simulink model "E33_VCU_simulink"  (R2014a)
settings: Solver=FixedStepDiscrete  StartTime=0.0  StopTime=10.0  FixedStep=0.0005  RelTol=1e-3
values from neighbouring files (symbols this model uses):
  Accu_FAN_Test = ecucoder_cal(Accu_FAN_Test)    [E33_VCU.m]
  Accu_FAN_threshold = ecucoder_cal(Accu_FAN_threshold)    [E33_VCU.m]
  APPS1_Voltage = ecucoder_cal(APPS1_Voltage)    [E33_VCU.m]
  APPS2_Voltage = ecucoder_cal(APPS2_Voltage)    [E33_VCU.m]
  APPS_Map = [0,1000]    [E33_VCU.m]
  APPS_threshold = ecucoder_cal(APPS_threshold)    [E33_VCU.m]
  Beep_Time = ecucoder_cal(Beep_Time)    [E33_VCU.m]
  BeeperTest = ecucoder_cal(BeeperTest)    [E33_VCU.m]
  BMSLedTest = ecucoder_cal(BMSLedTest)    [E33_VCU.m]
  BP_F_threshold = ecucoder_cal(BP_F_threshold)    [E33_VCU.m]
  BP_F_Voltage = ecucoder_cal(BP_F_Voltage)    [E33_VCU.m]
  BP_Map = [0,1000]    [E33_VCU.m]
  BP_R_Voltage = ecucoder_cal(BP_R_Voltage)    [E33_VCU.m]
  Brk_luminance = ecucoder_cal(Brk_luminance)    [E33_VCU.m]
  DCDC_Relay_Test = ecucoder_cal(DCDC_Relay_Test)    [E33_VCU.m]
  FactoryTestEnable = ecucoder_cal(FactoryTestEnable)    [E33_VCU.m]
  HardBrk_luminance = ecucoder_cal(HardBrk_luminance)    [E33_VCU.m]
  IMDLedTest = ecucoder_cal(IMDLedTest)    [E33_VCU.m]
  linear_FL_Map = ecucoder_cal(linear_FL_Map)    [E33_VCU.m]
  linear_FR_Map = ecucoder_cal(linear_FR_Map)    [E33_VCU.m]
  linear_Map = ecucoder_cal(linear_Map)    [E33_VCU.m]
  linear_RL_Map = ecucoder_cal(linear_RL_Map)    [E33_VCU.m]
  linear_RR_Map = ecucoder_cal(linear_RR_Map)    [E33_VCU.m]
  MaxPow = 40    [E33_VCU.m]
  MaxRPM = 5400    [E33_VCU.m]
  MaxRPMchangePerSec = ecucoder_cal(MaxRPMchangePerSec)    [E33_VCU.m]
  MaxTorqChangePerSec = ecucoder_cal(MaxTorqChangePerSec)    [E33_VCU.m]
  Motor_RPM_Map = (0:ceil(MaxRPM/100))*100    [E33_VCU.m]
  Pump_Test = ecucoder_cal(Pump_Test)    [E33_VCU.m]
  Pump_threshold = ecucoder_cal(Pump_threshold)    [E33_VCU.m]
  R2D_Light_Test = ecucoder_cal(R2D_Light_Test)    [E33_VCU.m]
  Radiator_FAN_Test = ecucoder_cal(Radiator_FAN_Test)    [E33_VCU.m]
  SCS_Error_5V = ecucoder_cal(SCS_Error_5V)    [E33_VCU.m]
  SCS_Error_GND = ecucoder_cal(SCS_Error_GND)    [E33_VCU.m]
  SPD_Coef = 1884/40    (= 47.1)    [E33_VCU.m]
  Tail_Light_Test = ecucoder_cal(Tail_Light_Test)    [E33_VCU.m]
  Tmanage_Map = [0,100]    [E33_VCU.m]
  Torq_percentage_Map = Motor_Torq_MAP/MaxTorq*1000    [E33_VCU.m]
libraries: simulink x164, ec55xxlib x44, dspswit3 x6
(part 4 of 5)

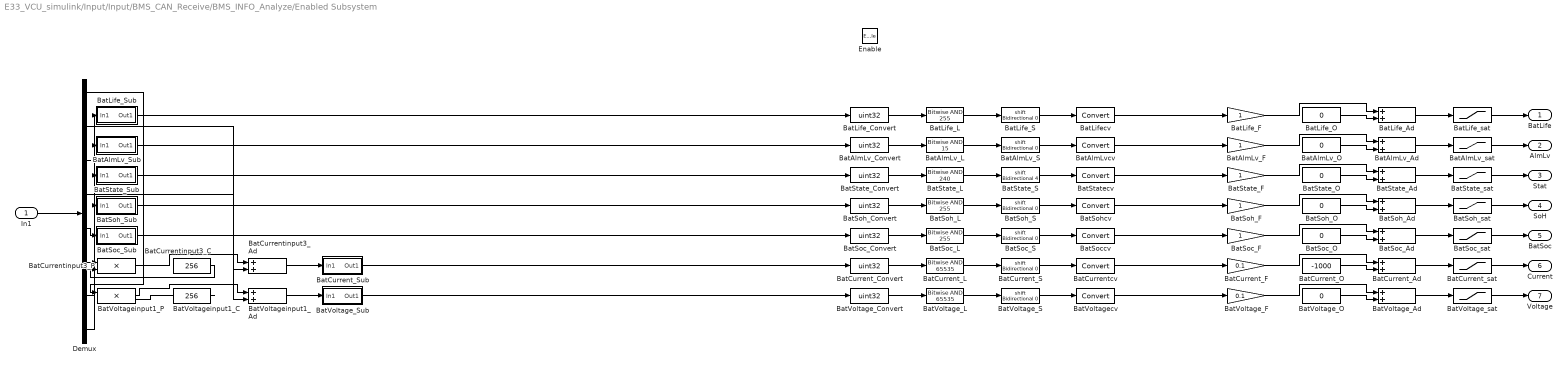
== system E33_VCU_simulink/Input/Input/BMS_CAN_Receive/BMS_INFO_Analyze/Enabled Subsystem ==
  In1 : Inport
  Enable : EnablePort
  BatAlmLv_Ad : Sum
  BatAlmLv_Convert : DataTypeConversion  OutDataTypeStr=uint32
  BatAlmLv_F : Gain
  BatAlmLv_L : simulink/Logic and Bit Operations/Bitwise Operator  logicop=AND  UseBitMask=on  BitMask=15  BitMaskRealWorld=Stored Integer
  BatAlmLv_O : Constant  Value=0  OutDataTypeStr=single
  BatAlmLv_S : ArithShift
  BatAlmLv_Sub : Subsystem
  BatAlmLv_sat : Saturate  UpperLimit=4  LowerLimit=0
  BatAlmLvcv : DataTypeConversion
  BatCurrent_Ad : Sum
  BatCurrent_Convert : DataTypeConversion  OutDataTypeStr=uint32
  BatCurrent_F : Gain  Gain=0.1
  BatCurrent_L : simulink/Logic and Bit Operations/Bitwise Operator  logicop=AND  UseBitMask=on  BitMask=65535  BitMaskRealWorld=Stored Integer
  BatCurrent_O : Constant  Value=-1000  OutDataTypeStr=single
  BatCurrent_S : ArithShift
  BatCurrent_Sub : Subsystem
  BatCurrent_sat : Saturate  UpperLimit=1000  LowerLimit=-1000
  BatCurrentcv : DataTypeConversion
  BatCurrentinput3_Ad : Sum
  BatCurrentinput3_C : Constant  Value=256
  BatCurrentinput3_P : Product
  BatLife_Ad : Sum
  BatLife_Convert : DataTypeConversion  OutDataTypeStr=uint32
  BatLife_F : Gain
  BatLife_L : simulink/Logic and Bit Operations/Bitwise Operator  logicop=AND  UseBitMask=on  BitMask=255  BitMaskRealWorld=Stored Integer
  BatLife_O : Constant  Value=0  OutDataTypeStr=single
  BatLife_S : ArithShift
  BatLife_Sub : Subsystem
  BatLife_sat : Saturate  UpperLimit=255  LowerLimit=0
  BatLifecv : DataTypeConversion
  BatSoc_Ad : Sum
  BatSoc_Convert : DataTypeConversion  OutDataTypeStr=uint32
  BatSoc_F : Gain
  BatSoc_L : simulink/Logic and Bit Operations/Bitwise Operator  logicop=AND  UseBitMask=on  BitMask=255  BitMaskRealWorld=Stored Integer
  BatSoc_O : Constant  Value=0  OutDataTypeStr=single
  BatSoc_S : ArithShift
  BatSoc_Sub : Subsystem
  BatSoc_sat : Saturate  UpperLimit=100  LowerLimit=0
  BatSoccv : DataTypeConversion
  BatSoh_Ad : Sum
  BatSoh_Convert : DataTypeConversion  OutDataTypeStr=uint32
  BatSoh_F : Gain
  BatSoh_L : simulink/Logic and Bit Operations/Bitwise Operator  logicop=AND  UseBitMask=on  BitMask=255  BitMaskRealWorld=Stored Integer
  BatSoh_O : Constant  Value=0  OutDataTypeStr=single
  BatSoh_S : ArithShift
  BatSoh_Sub : Subsystem
  BatSoh_sat : Saturate  UpperLimit=100  LowerLimit=0
  BatSohcv : DataTypeConversion
  BatState_Ad : Sum
  BatState_Convert : DataTypeConversion  OutDataTypeStr=uint32
  BatState_F : Gain
  BatState_L : simulink/Logic and Bit Operations/Bitwise Operator  logicop=AND  UseBitMask=on  BitMask=240  BitMaskRealWorld=Stored Integer
  BatState_O : Constant  Value=0  OutDataTypeStr=single
  BatState_S : ArithShift  BitShiftNumber=4
  BatState_Sub : Subsystem
  BatState_sat : Saturate  UpperLimit=7  LowerLimit=0
  BatStatecv : DataTypeConversion
  BatVoltage_Ad : Sum
  BatVoltage_Convert : DataTypeConversion  OutDataTypeStr=uint32
  BatVoltage_F : Gain  Gain=0.1
  BatVoltage_L : simulink/Logic and Bit Operations/Bitwise Operator  logicop=AND  UseBitMask=on  BitMask=65535  BitMaskRealWorld=Stored Integer
  BatVoltage_O : Constant  Value=0  OutDataTypeStr=single
  BatVoltage_S : ArithShift
  BatVoltage_Sub : Subsystem
  BatVoltage_sat : Saturate  UpperLimit=900  LowerLimit=0
  BatVoltagecv : DataTypeConversion
  BatVoltageinput1_Ad : Sum
  BatVoltageinput1_C : Constant  Value=256
  BatVoltageinput1_P : Product
  Demux : Demux  Outputs=8
  BatLife : Outport
  AlmLv : Outport  Port=2
  Stat : Outport  Port=3
  SoH : Outport  Port=4
  BatSoc : Outport  Port=5
  Current : Outport  Port=6
  Voltage : Outport  Port=7
  wires:
  In1/1 -> Demux/1
  BatVoltagecv/1 -> BatVoltage_F/1
  BatVoltage_S/1 -> BatVoltagecv/1
  BatVoltage_L/1 -> BatVoltage_S/1
  BatVoltage_Convert/1 -> BatVoltage_L/1
  BatVoltage_Sub/1(Out1) -> BatVoltage_Convert/1
  BatVoltageinput1_Ad/1 -> BatVoltage_Sub/1(In1)
  Demux/2 -> BatVoltageinput1_Ad/2
  BatVoltageinput1_P/1 -> BatVoltageinput1_Ad/1
  BatVoltageinput1_C/1 -> BatVoltageinput1_P/2
  Demux/1 -> BatVoltageinput1_P/1
  BatVoltage_sat/1 -> Voltage/1
  BatVoltage_Ad/1 -> BatVoltage_sat/1
  BatVoltage_O/1 -> BatVoltage_Ad/2
  BatVoltage_F/1 -> BatVoltage_Ad/1
  BatCurrentcv/1 -> BatCurrent_F/1
  BatCurrent_S/1 -> BatCurrentcv/1
  BatCurrent_L/1 -> BatCurrent_S/1
  BatCurrent_Convert/1 -> BatCurrent_L/1
  BatCurrent_Sub/1(Out1) -> BatCurrent_Convert/1
  BatCurrentinput3_Ad/1 -> BatCurrent_Sub/1(In1)
  Demux/4 -> BatCurrentinput3_Ad/2
  BatCurrentinput3_P/1 -> BatCurrentinput3_Ad/1
  BatCurrentinput3_C/1 -> BatCurrentinput3_P/2
  Demux/3 -> BatCurrentinput3_P/1
  BatCurrent_sat/1 -> Current/1
  BatCurrent_Ad/1 -> BatCurrent_sat/1
  BatCurrent_O/1 -> BatCurrent_Ad/2
  BatCurrent_F/1 -> BatCurrent_Ad/1
  BatSoccv/1 -> BatSoc_F/1
  BatSoc_S/1 -> BatSoccv/1
  BatSoc_L/1 -> BatSoc_S/1
  BatSoc_Convert/1 -> BatSoc_L/1
  BatSoc_Sub/1(Out1) -> BatSoc_Convert/1
  Demux/5 -> BatSoc_Sub/1(In1)
  BatSoc_sat/1 -> BatSoc/1
  BatSoc_Ad/1 -> BatSoc_sat/1
  BatSoc_O/1 -> BatSoc_Ad/2
  BatSoc_F/1 -> BatSoc_Ad/1
  BatSohcv/1 -> BatSoh_F/1
  BatSoh_S/1 -> BatSohcv/1
  BatSoh_L/1 -> BatSoh_S/1
  BatSoh_Convert/1 -> BatSoh_L/1
  BatSoh_Sub/1(Out1) -> BatSoh_Convert/1
  Demux/6 -> BatSoh_Sub/1(In1)
  BatSoh_sat/1 -> SoH/1
  BatSoh_Ad/1 -> BatSoh_sat/1
  BatSoh_O/1 -> BatSoh_Ad/2
  BatSoh_F/1 -> BatSoh_Ad/1
  BatStatecv/1 -> BatState_F/1
  BatState_S/1 -> BatStatecv/1
  BatState_L/1 -> BatState_S/1
  BatState_Convert/1 -> BatState_L/1
  BatState_Sub/1(Out1) -> BatState_Convert/1
  BatState_sat/1 -> Stat/1
  BatState_Ad/1 -> BatState_sat/1
  BatState_O/1 -> BatState_Ad/2
  BatState_F/1 -> BatState_Ad/1
  BatAlmLvcv/1 -> BatAlmLv_F/1
  BatAlmLv_S/1 -> BatAlmLvcv/1
  BatAlmLv_L/1 -> BatAlmLv_S/1
  BatAlmLv_Convert/1 -> BatAlmLv_L/1
  BatAlmLv_Sub/1(Out1) -> BatAlmLv_Convert/1
  Demux/7 -> BatAlmLv_Sub/1(In1), BatState_Sub/1(In1)
  BatAlmLv_sat/1 -> AlmLv/1
  BatAlmLv_Ad/1 -> BatAlmLv_sat/1
  BatAlmLv_O/1 -> BatAlmLv_Ad/2
  BatAlmLv_F/1 -> BatAlmLv_Ad/1
  BatLifecv/1 -> BatLife_F/1
  BatLife_S/1 -> BatLifecv/1
  BatLife_L/1 -> BatLife_S/1
  BatLife_Convert/1 -> BatLife_L/1
  BatLife_Sub/1(Out1) -> BatLife_Convert/1
  Demux/8 -> BatLife_Sub/1(In1)
  BatLife_sat/1 -> BatLife/1
  BatLife_Ad/1 -> BatLife_sat/1
  BatLife_O/1 -> BatLife_Ad/2
  BatLife_F/1 -> BatLife_Ad/1

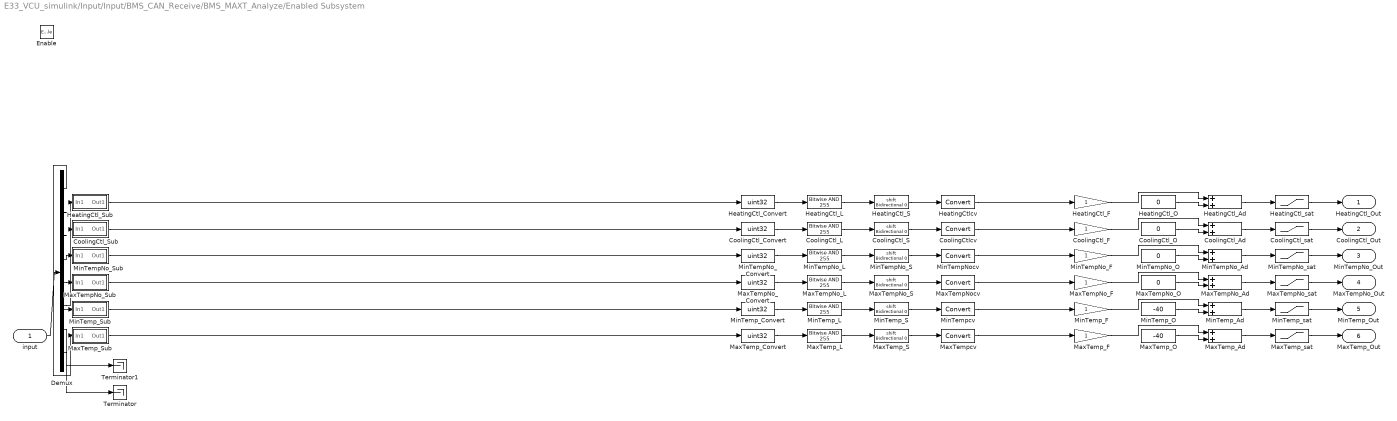
== system E33_VCU_simulink/Input/Input/BMS_CAN_Receive/BMS_MAXT_Analyze/Enabled Subsystem ==
  input : Inport
  Enable : EnablePort
  CoolingCtl_Ad : Sum
  CoolingCtl_Convert : DataTypeConversion  OutDataTypeStr=uint32
  CoolingCtl_F : Gain
  CoolingCtl_L : simulink/Logic and Bit Operations/Bitwise Operator  logicop=AND  UseBitMask=on  BitMask=255  BitMaskRealWorld=Stored Integer
  CoolingCtl_O : Constant  Value=0  OutDataTypeStr=single
  CoolingCtl_S : ArithShift
  CoolingCtl_Sub : Subsystem
  CoolingCtl_sat : Saturate  UpperLimit=1  LowerLimit=0
  CoolingCtlcv : DataTypeConversion
  Demux : Demux  Outputs=8
  HeatingCtl_Ad : Sum
  HeatingCtl_Convert : DataTypeConversion  OutDataTypeStr=uint32
  HeatingCtl_F : Gain
  HeatingCtl_L : simulink/Logic and Bit Operations/Bitwise Operator  logicop=AND  UseBitMask=on  BitMask=255  BitMaskRealWorld=Stored Integer
  HeatingCtl_O : Constant  Value=0  OutDataTypeStr=single
  HeatingCtl_S : ArithShift
  HeatingCtl_Sub : Subsystem
  HeatingCtl_sat : Saturate  UpperLimit=1  LowerLimit=0
  HeatingCtlcv : DataTypeConversion
  MaxTempNo_Ad : Sum
  MaxTempNo_Convert : DataTypeConversion  OutDataTypeStr=uint32
  MaxTempNo_F : Gain
  MaxTempNo_L : simulink/Logic and Bit Operations/Bitwise Operator  logicop=AND  UseBitMask=on  BitMask=255  BitMaskRealWorld=Stored Integer
  MaxTempNo_O : Constant  Value=0  OutDataTypeStr=single
  MaxTempNo_S : ArithShift
  MaxTempNo_Sub : Subsystem
  MaxTempNo_sat : Saturate  UpperLimit=255  LowerLimit=0
  MaxTempNocv : DataTypeConversion
  MaxTemp_Ad : Sum
  MaxTemp_Convert : DataTypeConversion  OutDataTypeStr=uint32
  MaxTemp_F : Gain
  MaxTemp_L : simulink/Logic and Bit Operations/Bitwise Operator  logicop=AND  UseBitMask=on  BitMask=255  BitMaskRealWorld=Stored Integer
  MaxTemp_O : Constant  Value=-40  OutDataTypeStr=single
  MaxTemp_S : ArithShift
  MaxTemp_Sub : Subsystem
  MaxTemp_sat : Saturate  UpperLimit=120  LowerLimit=-40
  MaxTempcv : DataTypeConversion
  MinTempNo_Ad : Sum
  MinTempNo_Convert : DataTypeConversion  OutDataTypeStr=uint32
  MinTempNo_F : Gain
  MinTempNo_L : simulink/Logic and Bit Operations/Bitwise Operator  logicop=AND  UseBitMask=on  BitMask=255  BitMaskRealWorld=Stored Integer
  MinTempNo_O : Constant  Value=0  OutDataTypeStr=single
  MinTempNo_S : ArithShift
  MinTempNo_Sub : Subsystem
  MinTempNo_sat : Saturate  UpperLimit=255  LowerLimit=0
  MinTempNocv : DataTypeConversion
  MinTemp_Ad : Sum
  MinTemp_Convert : DataTypeConversion  OutDataTypeStr=uint32
  MinTemp_F : Gain
  MinTemp_L : simulink/Logic and Bit Operations/Bitwise Operator  logicop=AND  UseBitMask=on  BitMask=255  BitMaskRealWorld=Stored Integer
  MinTemp_O : Constant  Value=-40  OutDataTypeStr=single
  MinTemp_S : ArithShift
  MinTemp_Sub : Subsystem
  MinTemp_sat : Saturate  UpperLimit=120  LowerLimit=-40
  MinTempcv : DataTypeConversion
  Terminator : Terminator
  Terminator1 : Terminator
  HeatingCtl_Out : Outport
  CoolingCtl_Out : Outport  Port=2
  MinTempNo_Out : Outport  Port=3
  MaxTempNo_Out : Outport  Port=4
  MinTemp_Out : Outport  Port=5
  MaxTemp_Out : Outport  Port=6
  wires:
  HeatingCtl_F/1 -> HeatingCtl_Ad/1
  HeatingCtl_O/1 -> HeatingCtl_Ad/2
  HeatingCtl_Ad/1 -> HeatingCtl_sat/1
  HeatingCtl_sat/1 -> HeatingCtl_Out/1
  Demux/6 -> HeatingCtl_Sub/1(In1)
  HeatingCtl_Sub/1(Out1) -> HeatingCtl_Convert/1
  HeatingCtl_Convert/1 -> HeatingCtl_L/1
  HeatingCtl_L/1 -> HeatingCtl_S/1
  HeatingCtl_S/1 -> HeatingCtlcv/1
  HeatingCtlcv/1 -> HeatingCtl_F/1
  CoolingCtl_F/1 -> CoolingCtl_Ad/1
  CoolingCtl_O/1 -> CoolingCtl_Ad/2
  CoolingCtl_Ad/1 -> CoolingCtl_sat/1
  CoolingCtl_sat/1 -> CoolingCtl_Out/1
  Demux/5 -> CoolingCtl_Sub/1(In1)
  CoolingCtl_Sub/1(Out1) -> CoolingCtl_Convert/1
  CoolingCtl_Convert/1 -> CoolingCtl_L/1
  CoolingCtl_L/1 -> CoolingCtl_S/1
  CoolingCtl_S/1 -> CoolingCtlcv/1
  CoolingCtlcv/1 -> CoolingCtl_F/1
  MinTempNo_F/1 -> MinTempNo_Ad/1
  MinTempNo_O/1 -> MinTempNo_Ad/2
  MinTempNo_Ad/1 -> MinTempNo_sat/1
  MinTempNo_sat/1 -> MinTempNo_Out/1
  Demux/4 -> MinTempNo_Sub/1(In1)
  MinTempNo_Sub/1(Out1) -> MinTempNo_Convert/1
  MinTempNo_Convert/1 -> MinTempNo_L/1
  MinTempNo_L/1 -> MinTempNo_S/1
  MinTempNo_S/1 -> MinTempNocv/1
  MinTempNocv/1 -> MinTempNo_F/1
  MaxTempNo_F/1 -> MaxTempNo_Ad/1
  MaxTempNo_O/1 -> MaxTempNo_Ad/2
  MaxTempNo_Ad/1 -> MaxTempNo_sat/1
  MaxTempNo_sat/1 -> MaxTempNo_Out/1
  Demux/3 -> MaxTempNo_Sub/1(In1)
  MaxTempNo_Sub/1(Out1) -> MaxTempNo_Convert/1
  MaxTempNo_Convert/1 -> MaxTempNo_L/1
  MaxTempNo_L/1 -> MaxTempNo_S/1
  MaxTempNo_S/1 -> MaxTempNocv/1
  MaxTempNocv/1 -> MaxTempNo_F/1
  MinTemp_F/1 -> MinTemp_Ad/1
  MinTemp_O/1 -> MinTemp_Ad/2
  MinTemp_Ad/1 -> MinTemp_sat/1
  MinTemp_sat/1 -> MinTemp_Out/1
  Demux/2 -> MinTemp_Sub/1(In1)
  MinTemp_Sub/1(Out1) -> MinTemp_Convert/1
  MinTemp_Convert/1 -> MinTemp_L/1
  MinTemp_L/1 -> MinTemp_S/1
  MinTemp_S/1 -> MinTempcv/1
  MinTempcv/1 -> MinTemp_F/1
  MaxTemp_F/1 -> MaxTemp_Ad/1
  MaxTemp_O/1 -> MaxTemp_Ad/2
  MaxTemp_Ad/1 -> MaxTemp_sat/1
  MaxTemp_sat/1 -> MaxTemp_Out/1
  Demux/1 -> MaxTemp_Sub/1(In1)
  MaxTemp_Sub/1(Out1) -> MaxTemp_Convert/1
  MaxTemp_Convert/1 -> MaxTemp_L/1
  MaxTemp_L/1 -> MaxTemp_S/1
  MaxTemp_S/1 -> MaxTempcv/1
  MaxTempcv/1 -> MaxTemp_F/1
  input/1 -> Demux/1
  Demux/7 -> Terminator/1
  Demux/8 -> Terminator1/1

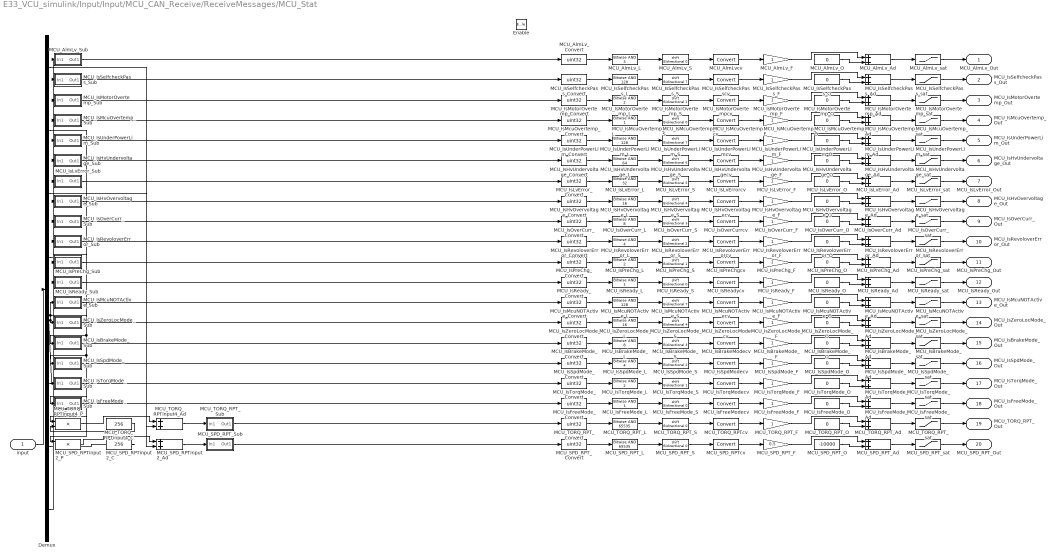
== system E33_VCU_simulink/Input/Input/MCU_CAN_Receive/ReceiveMessages/MCU_Stat ==
  input : Inport
  Enable : EnablePort
  Demux : Demux  Outputs=8
  MCU_AlmLv_Ad : Sum
  MCU_AlmLv_Convert : DataTypeConversion  OutDataTypeStr=uint32
  MCU_AlmLv_F : Gain
  MCU_AlmLv_L : simulink/Logic and Bit Operations/Bitwise Operator  logicop=AND  UseBitMask=on  BitMask=3  BitMaskRealWorld=Stored Integer
  MCU_AlmLv_O : Constant  Value=0  OutDataTypeStr=single
  MCU_AlmLv_S : ArithShift
  MCU_AlmLv_Sub : Subsystem
  MCU_AlmLv_sat : Saturate  UpperLimit=3  LowerLimit=0
  MCU_AlmLvcv : DataTypeConversion
  MCU_IsBrakeMode_Ad : Sum
  MCU_IsBrakeMode_Convert : DataTypeConversion  OutDataTypeStr=uint32
  MCU_IsBrakeMode_F : Gain
  MCU_IsBrakeMode_L : simulink/Logic and Bit Operations/Bitwise Operator  logicop=AND  UseBitMask=on  BitMask=8  BitMaskRealWorld=Stored Integer
  MCU_IsBrakeMode_O : Constant  Value=0  OutDataTypeStr=single
  MCU_IsBrakeMode_S : ArithShift  BitShiftNumber=3
  MCU_IsBrakeMode_Sub : Subsystem
  MCU_IsBrakeMode_sat : Saturate  UpperLimit=1  LowerLimit=0
  MCU_IsBrakeModecv : DataTypeConversion
  MCU_IsFreeMode_Ad : Sum
  MCU_IsFreeMode_Convert : DataTypeConversion  OutDataTypeStr=uint32
  MCU_IsFreeMode_F : Gain
  MCU_IsFreeMode_L : simulink/Logic and Bit Operations/Bitwise Operator  logicop=AND  UseBitMask=on  BitMask=1  BitMaskRealWorld=Stored Integer
  MCU_IsFreeMode_O : Constant  Value=0  OutDataTypeStr=single
  MCU_IsFreeMode_S : ArithShift
  MCU_IsFreeMode_Sub : Subsystem
  MCU_IsFreeMode_sat : Saturate  UpperLimit=1  LowerLimit=0
  MCU_IsFreeModecv : DataTypeConversion
  MCU_IsHvOvervoltage_Ad : Sum
  MCU_IsHvOvervoltage_Convert : DataTypeConversion  OutDataTypeStr=uint32
  MCU_IsHvOvervoltage_F : Gain
  MCU_IsHvOvervoltage_L : simulink/Logic and Bit Operations/Bitwise Operator  logicop=AND  UseBitMask=on  BitMask=16  BitMaskRealWorld=Stored Integer
  MCU_IsHvOvervoltage_O : Constant  Value=0  OutDataTypeStr=single
  MCU_IsHvOvervoltage_S : ArithShift  BitShiftNumber=4
  MCU_IsHvOvervoltage_Sub : Subsystem
  MCU_IsHvOvervoltage_sat : Saturate  UpperLimit=1  LowerLimit=0
  MCU_IsHvOvervoltagecv : DataTypeConversion
  MCU_IsHvUndervoltage_Ad : Sum
  MCU_IsHvUndervoltage_Convert : DataTypeConversion  OutDataTypeStr=uint32
  MCU_IsHvUndervoltage_F : Gain
  MCU_IsHvUndervoltage_L : simulink/Logic and Bit Operations/Bitwise Operator  logicop=AND  UseBitMask=on  BitMask=64  BitMaskRealWorld=Stored Integer
  MCU_IsHvUndervoltage_O : Constant  Value=0  OutDataTypeStr=single
  MCU_IsHvUndervoltage_S : ArithShift  BitShiftNumber=6
  MCU_IsHvUndervoltage_Sub : Subsystem
  MCU_IsHvUndervoltage_sat : Saturate  UpperLimit=1  LowerLimit=0
  MCU_IsHvUndervoltagecv : DataTypeConversion
  MCU_IsLvError_Ad : Sum
  MCU_IsLvError_Convert : DataTypeConversion  OutDataTypeStr=uint32
  MCU_IsLvError_F : Gain
  MCU_IsLvError_L : simulink/Logic and Bit Operations/Bitwise Operator  logicop=AND  UseBitMask=on  BitMask=32  BitMaskRealWorld=Stored Integer
  MCU_IsLvError_O : Constant  Value=0  OutDataTypeStr=single
  MCU_IsLvError_S : ArithShift  BitShiftNumber=5
  MCU_IsLvError_Sub : Subsystem
  MCU_IsLvError_sat : Saturate  UpperLimit=1  LowerLimit=0
  MCU_IsLvErrorcv : DataTypeConversion
  MCU_IsMcuNOTActive_Ad : Sum
  MCU_IsMcuNOTActive_Convert : DataTypeConversion  OutDataTypeStr=uint32
  MCU_IsMcuNOTActive_F : Gain
  MCU_IsMcuNOTActive_L : simulink/Logic and Bit Operations/Bitwise Operator  logicop=AND  UseBitMask=on  BitMask=128  BitMaskRealWorld=Stored Integer
  MCU_IsMcuNOTActive_O : Constant  Value=0  OutDataTypeStr=single
  MCU_IsMcuNOTActive_S : ArithShift  BitShiftNumber=7
  MCU_IsMcuNOTActive_Sub : Subsystem
  MCU_IsMcuNOTActive_sat : Saturate  UpperLimit=1  LowerLimit=0
  MCU_IsMcuNOTActivecv : DataTypeConversion
  MCU_IsMcuOvertemp_Ad : Sum
  MCU_IsMcuOvertemp_Convert : DataTypeConversion  OutDataTypeStr=uint32
  MCU_IsMcuOvertemp_F : Gain
  MCU_IsMcuOvertemp_L : simulink/Logic and Bit Operations/Bitwise Operator  logicop=AND  UseBitMask=on  BitMask=1  BitMaskRealWorld=Stored Integer
  MCU_IsMcuOvertemp_O : Constant  Value=0  OutDataTypeStr=single
  MCU_IsMcuOvertemp_S : ArithShift
  MCU_IsMcuOvertemp_Sub : Subsystem
  MCU_IsMcuOvertemp_sat : Saturate  UpperLimit=1  LowerLimit=0
  MCU_IsMcuOvertempcv : DataTypeConversion
  MCU_IsMotorOvertemp_Ad : Sum
  MCU_IsMotorOvertemp_Convert : DataTypeConversion  OutDataTypeStr=uint32
  MCU_IsMotorOvertemp_F : Gain
  MCU_IsMotorOvertemp_L : simulink/Logic and Bit Operations/Bitwise Operator  logicop=AND  UseBitMask=on  BitMask=2  BitMaskRealWorld=Stored Integer
  MCU_IsMotorOvertemp_O : Constant  Value=0  OutDataTypeStr=single
  MCU_IsMotorOvertemp_S : ArithShift  BitShiftNumber=1
  MCU_IsMotorOvertemp_Sub : Subsystem
  MCU_IsMotorOvertemp_sat : Saturate  UpperLimit=1  LowerLimit=0
  MCU_IsMotorOvertempcv : DataTypeConversion
  MCU_IsOverCurr_Ad : Sum
  MCU_IsOverCurr_Convert : DataTypeConversion  OutDataTypeStr=uint32
  MCU_IsOverCurr_F : Gain
  MCU_IsOverCurr_L : simulink/Logic and Bit Operations/Bitwise Operator  logicop=AND  UseBitMask=on  BitMask=8  BitMaskRealWorld=Stored Integer
  MCU_IsOverCurr_O : Constant  Value=0  OutDataTypeStr=single
  MCU_IsOverCurr_S : ArithShift  BitShiftNumber=3
  MCU_IsOverCurr_Sub : Subsystem
  MCU_IsOverCurr_sat : Saturate  UpperLimit=1  LowerLimit=0
  MCU_IsOverCurrcv : DataTypeConversion
  MCU_IsPreChg_Ad : Sum
  MCU_IsPreChg_Convert : DataTypeConversion  OutDataTypeStr=uint32
  MCU_IsPreChg_F : Gain
  MCU_IsPreChg_L : simulink/Logic and Bit Operations/Bitwise Operator  logicop=AND  UseBitMask=on  BitMask=2  BitMaskRealWorld=Stored Integer
  MCU_IsPreChg_O : Constant  Value=0  OutDataTypeStr=single
  MCU_IsPreChg_S : ArithShift  BitShiftNumber=1
  MCU_IsPreChg_Sub : Subsystem
  MCU_IsPreChg_sat : Saturate  UpperLimit=255  LowerLimit=0
  MCU_IsPreChgcv : DataTypeConversion
  MCU_IsReady_Ad : Sum
  MCU_IsReady_Convert : DataTypeConversion  OutDataTypeStr=uint32
  MCU_IsReady_F : Gain
  MCU_IsReady_L : simulink/Logic and Bit Operations/Bitwise Operator  logicop=AND  UseBitMask=on  BitMask=1  BitMaskRealWorld=Stored Integer
  MCU_IsReady_O : Constant  Value=0  OutDataTypeStr=single
  MCU_IsReady_S : ArithShift
  MCU_IsReady_Sub : Subsystem
  MCU_IsReady_sat : Saturate  UpperLimit=1  LowerLimit=0
  MCU_IsReadycv : DataTypeConversion
  MCU_IsRevoloverError_Ad : Sum
  MCU_IsRevoloverError_Convert : DataTypeConversion  OutDataTypeStr=uint32
  MCU_IsRevoloverError_F : Gain
  MCU_IsRevoloverError_L : simulink/Logic and Bit Operations/Bitwise Operator  logicop=AND  UseBitMask=on  BitMask=4  BitMaskRealWorld=Stored Integer
  MCU_IsRevoloverError_O : Constant  Value=0  OutDataTypeStr=single
  MCU_IsRevoloverError_S : ArithShift  BitShiftNumber=2
  MCU_IsRevoloverError_Sub : Subsystem
  MCU_IsRevoloverError_sat : Saturate  UpperLimit=1  LowerLimit=0
  MCU_IsRevoloverErrorcv : DataTypeConversion
  MCU_IsSelfcheckPass_Ad : Sum
  MCU_IsSelfcheckPass_Convert : DataTypeConversion  OutDataTypeStr=uint32
  MCU_IsSelfcheckPass_F : Gain
  MCU_IsSelfcheckPass_L : simulink/Logic and Bit Operations/Bitwise Operator  logicop=AND  UseBitMask=on  BitMask=128  BitMaskRealWorld=Stored Integer
  MCU_IsSelfcheckPass_O : Constant  Value=0  OutDataTypeStr=single
  MCU_IsSelfcheckPass_S : ArithShift  BitShiftNumber=7
  MCU_IsSelfcheckPass_Sub : Subsystem
  MCU_IsSelfcheckPass_sat : Saturate  UpperLimit=1  LowerLimit=0
  MCU_IsSelfcheckPasscv : DataTypeConversion
  MCU_IsSpdMode_Ad : Sum
  MCU_IsSpdMode_Convert : DataTypeConversion  OutDataTypeStr=uint32
  MCU_IsSpdMode_F : Gain
  MCU_IsSpdMode_L : simulink/Logic and Bit Operations/Bitwise Operator  logicop=AND  UseBitMask=on  BitMask=4  BitMaskRealWorld=Stored Integer
  MCU_IsSpdMode_O : Constant  Value=0  OutDataTypeStr=single
  MCU_IsSpdMode_S : ArithShift  BitShiftNumber=2
  MCU_IsSpdMode_Sub : Subsystem
  MCU_IsSpdMode_sat : Saturate  UpperLimit=1  LowerLimit=0
  MCU_IsSpdModecv : DataTypeConversion
  MCU_IsTorqMode_Ad : Sum
  MCU_IsTorqMode_Convert : DataTypeConversion  OutDataTypeStr=uint32
  MCU_IsTorqMode_F : Gain
  MCU_IsTorqMode_L : simulink/Logic and Bit Operations/Bitwise Operator  logicop=AND  UseBitMask=on  BitMask=2  BitMaskRealWorld=Stored Integer
  MCU_IsTorqMode_O : Constant  Value=0  OutDataTypeStr=single
  MCU_IsTorqMode_S : ArithShift  BitShiftNumber=1
  MCU_IsTorqMode_Sub : Subsystem
  MCU_IsTorqMode_sat : Saturate  UpperLimit=1  LowerLimit=0
  MCU_IsTorqModecv : DataTypeConversion
  MCU_IsUnderPowerLim_Ad : Sum
  MCU_IsUnderPowerLim_Convert : DataTypeConversion  OutDataTypeStr=uint32
  MCU_IsUnderPowerLim_F : Gain
  MCU_IsUnderPowerLim_L : simulink/Logic and Bit Operations/Bitwise Operator  logicop=AND  UseBitMask=on  BitMask=128  BitMaskRealWorld=Stored Integer
  MCU_IsUnderPowerLim_O : Constant  Value=0  OutDataTypeStr=single
  MCU_IsUnderPowerLim_S : ArithShift  BitShiftNumber=7
  MCU_IsUnderPowerLim_Sub : Subsystem
  MCU_IsUnderPowerLim_sat : Saturate  UpperLimit=1  LowerLimit=0
  MCU_IsUnderPowerLimcv : DataTypeConversion
  MCU_IsZeroLocMode_Ad : Sum
  MCU_IsZeroLocMode_Convert : DataTypeConversion  OutDataTypeStr=uint32
  MCU_IsZeroLocMode_F : Gain
  MCU_IsZeroLocMode_L : simulink/Logic and Bit Operations/Bitwise Operator  logicop=AND  UseBitMask=on  BitMask=16  BitMaskRealWorld=Stored Integer
  MCU_IsZeroLocMode_O : Constant  Value=0  OutDataTypeStr=single
  MCU_IsZeroLocMode_S : ArithShift  BitShiftNumber=4
  MCU_IsZeroLocMode_Sub : Subsystem
  MCU_IsZeroLocMode_sat : Saturate  UpperLimit=1  LowerLimit=0
  MCU_IsZeroLocModecv : DataTypeConversion
  MCU_SPD_RPT_Ad : Sum
  MCU_SPD_RPT_Convert : DataTypeConversion  OutDataTypeStr=uint32
  MCU_SPD_RPT_F : Gain  Gain=0.5
  MCU_SPD_RPT_L : simulink/Logic and Bit Operations/Bitwise Operator  logicop=AND  UseBitMask=on  BitMask=65535  BitMaskRealWorld=Stored Integer
  MCU_SPD_RPT_O : Constant  Value=-10000  OutDataTypeStr=single
  MCU_SPD_RPT_S : ArithShift
  MCU_SPD_RPT_Sub : Subsystem
  MCU_SPD_RPT_sat : Saturate  UpperLimit=10000  LowerLimit=-10000
  MCU_SPD_RPTcv : DataTypeConversion
  MCU_SPD_RPTinput2_Ad : Sum
  MCU_SPD_RPTinput2_C : Constant  Value=256
  MCU_SPD_RPTinput2_P : Product
  MCU_TORQ_RPT_Ad : Sum
  MCU_TORQ_RPT_Convert : DataTypeConversion  OutDataTypeStr=uint32
  MCU_TORQ_RPT_F : Gain
  MCU_TORQ_RPT_L : simulink/Logic and Bit Operations/Bitwise Operator  logicop=AND  UseBitMask=on  BitMask=65535  BitMaskRealWorld=Stored Integer
  MCU_TORQ_RPT_O : Constant  Value=0  OutDataTypeStr=single
  MCU_TORQ_RPT_S : ArithShift
  MCU_TORQ_RPT_Sub : Subsystem
  MCU_TORQ_RPT_sat : Saturate  UpperLimit=1000  LowerLimit=0
  MCU_TORQ_RPTcv : DataTypeConversion
  MCU_TORQ_RPTinput4_Ad : Sum
  MCU_TORQ_RPTinput4_C : Constant  Value=256
  MCU_TORQ_RPTinput4_P : Product
  MCU_AlmLv_Out : Outport
  MCU_IsSelfcheckPass_Out : Outport  Port=2
  MCU_IsMotorOvertemp_Out : Outport  Port=3
  MCU_IsMcuOvertemp_Out : Outport  Port=4
  MCU_IsUnderPowerLim_Out : Outport  Port=5
  MCU_IsHvUndervoltage_Out : Outport  Port=6
  MCU_IsLvError_Out : Outport  Port=7
  MCU_IsHvOvervoltage_Out : Outport  Port=8
  MCU_IsOverCurr_Out : Outport  Port=9
  MCU_IsRevoloverError_Out : Outport  Port=10
  MCU_IsPreChg_Out : Outport  Port=11
  MCU_IsReady_Out : Outport  Port=12
  MCU_IsMcuNOTActive_Out : Outport  Port=13
  MCU_IsZeroLocMode_Out : Outport  Port=14
  MCU_IsBrakeMode_Out : Outport  Port=15
  MCU_IsSpdMode_Out : Outport  Port=16
  MCU_IsTorqMode_Out : Outport  Port=17
  MCU_IsFreeMode_Out : Outport  Port=18
  MCU_TORQ_RPT_Out : Outport  Port=19
  MCU_SPD_RPT_Out : Outport  Port=20
  wires:
  input/1 -> Demux/1
  MCU_SPD_RPTcv/1 -> MCU_SPD_RPT_F/1
  MCU_SPD_RPT_S/1 -> MCU_SPD_RPTcv/1
  MCU_SPD_RPT_L/1 -> MCU_SPD_RPT_S/1
  MCU_SPD_RPT_Convert/1 -> MCU_SPD_RPT_L/1
  MCU_SPD_RPT_Sub/1(Out1) -> MCU_SPD_RPT_Convert/1
  MCU_SPD_RPTinput2_Ad/1 -> MCU_SPD_RPT_Sub/1(In1)
  Demux/1 -> MCU_SPD_RPTinput2_Ad/2
  MCU_SPD_RPTinput2_P/1 -> MCU_SPD_RPTinput2_Ad/1
  MCU_SPD_RPTinput2_C/1 -> MCU_SPD_RPTinput2_P/2
  Demux/2 -> MCU_SPD_RPTinput2_P/1
  MCU_SPD_RPT_sat/1 -> MCU_SPD_RPT_Out/1
  MCU_SPD_RPT_Ad/1 -> MCU_SPD_RPT_sat/1
  MCU_SPD_RPT_O/1 -> MCU_SPD_RPT_Ad/2
  MCU_SPD_RPT_F/1 -> MCU_SPD_RPT_Ad/1
  MCU_TORQ_RPTcv/1 -> MCU_TORQ_RPT_F/1
  MCU_TORQ_RPT_S/1 -> MCU_TORQ_RPTcv/1
  MCU_TORQ_RPT_L/1 -> MCU_TORQ_RPT_S/1
  MCU_TORQ_RPT_Convert/1 -> MCU_TORQ_RPT_L/1
  MCU_TORQ_RPT_Sub/1(Out1) -> MCU_TORQ_RPT_Convert/1
  MCU_TORQ_RPTinput4_Ad/1 -> MCU_TORQ_RPT_Sub/1(In1)
  Demux/3 -> MCU_TORQ_RPTinput4_Ad/2
  MCU_TORQ_RPTinput4_P/1 -> MCU_TORQ_RPTinput4_Ad/1
  MCU_TORQ_RPTinput4_C/1 -> MCU_TORQ_RPTinput4_P/2
  Demux/4 -> MCU_TORQ_RPTinput4_P/1
  MCU_TORQ_RPT_sat/1 -> MCU_TORQ_RPT_Out/1
  MCU_TORQ_RPT_Ad/1 -> MCU_TORQ_RPT_sat/1
  MCU_TORQ_RPT_O/1 -> MCU_TORQ_RPT_Ad/2
  MCU_TORQ_RPT_F/1 -> MCU_TORQ_RPT_Ad/1
  MCU_IsFreeModecv/1 -> MCU_IsFreeMode_F/1
  MCU_IsFreeMode_S/1 -> MCU_IsFreeModecv/1
  MCU_IsFreeMode_L/1 -> MCU_IsFreeMode_S/1
  MCU_IsFreeMode_Convert/1 -> MCU_IsFreeMode_L/1
  MCU_IsFreeMode_Sub/1(Out1) -> MCU_IsFreeMode_Convert/1
  MCU_IsFreeMode_sat/1 -> MCU_IsFreeMode_Out/1
  MCU_IsFreeMode_Ad/1 -> MCU_IsFreeMode_sat/1
  MCU_IsFreeMode_O/1 -> MCU_IsFreeMode_Ad/2
  MCU_IsFreeMode_F/1 -> MCU_IsFreeMode_Ad/1
  MCU_IsTorqModecv/1 -> MCU_IsTorqMode_F/1
  MCU_IsTorqMode_S/1 -> MCU_IsTorqModecv/1
  MCU_IsTorqMode_L/1 -> MCU_IsTorqMode_S/1
  MCU_IsTorqMode_Convert/1 -> MCU_IsTorqMode_L/1
  MCU_IsTorqMode_Sub/1(Out1) -> MCU_IsTorqMode_Convert/1
  MCU_IsTorqMode_sat/1 -> MCU_IsTorqMode_Out/1
  MCU_IsTorqMode_Ad/1 -> MCU_IsTorqMode_sat/1
  MCU_IsTorqMode_O/1 -> MCU_IsTorqMode_Ad/2
  MCU_IsTorqMode_F/1 -> MCU_IsTorqMode_Ad/1
  MCU_IsSpdModecv/1 -> MCU_IsSpdMode_F/1
  MCU_IsSpdMode_S/1 -> MCU_IsSpdModecv/1
  MCU_IsSpdMode_L/1 -> MCU_IsSpdMode_S/1
  MCU_IsSpdMode_Convert/1 -> MCU_IsSpdMode_L/1
  MCU_IsSpdMode_Sub/1(Out1) -> MCU_IsSpdMode_Convert/1
  MCU_IsSpdMode_sat/1 -> MCU_IsSpdMode_Out/1
  MCU_IsSpdMode_Ad/1 -> MCU_IsSpdMode_sat/1
  MCU_IsSpdMode_O/1 -> MCU_IsSpdMode_Ad/2
  MCU_IsSpdMode_F/1 -> MCU_IsSpdMode_Ad/1
  MCU_IsBrakeModecv/1 -> MCU_IsBrakeMode_F/1
  MCU_IsBrakeMode_S/1 -> MCU_IsBrakeModecv/1
  MCU_IsBrakeMode_L/1 -> MCU_IsBrakeMode_S/1
  MCU_IsBrakeMode_Convert/1 -> MCU_IsBrakeMode_L/1
  MCU_IsBrakeMode_Sub/1(Out1) -> MCU_IsBrakeMode_Convert/1
  MCU_IsBrakeMode_sat/1 -> MCU_IsBrakeMode_Out/1
  MCU_IsBrakeMode_Ad/1 -> MCU_IsBrakeMode_sat/1
  MCU_IsBrakeMode_O/1 -> MCU_IsBrakeMode_Ad/2
  MCU_IsBrakeMode_F/1 -> MCU_IsBrakeMode_Ad/1
  MCU_IsZeroLocModecv/1 -> MCU_IsZeroLocMode_F/1
  MCU_IsZeroLocMode_S/1 -> MCU_IsZeroLocModecv/1
  MCU_IsZeroLocMode_L/1 -> MCU_IsZeroLocMode_S/1
  MCU_IsZeroLocMode_Convert/1 -> MCU_IsZeroLocMode_L/1
  MCU_IsZeroLocMode_Sub/1(Out1) -> MCU_IsZeroLocMode_Convert/1
  MCU_IsZeroLocMode_sat/1 -> MCU_IsZeroLocMode_Out/1
  MCU_IsZeroLocMode_Ad/1 -> MCU_IsZeroLocMode_sat/1
  MCU_IsZeroLocMode_O/1 -> MCU_IsZeroLocMode_Ad/2
  MCU_IsZeroLocMode_F/1 -> MCU_IsZeroLocMode_Ad/1
  MCU_IsMcuNOTActivecv/1 -> MCU_IsMcuNOTActive_F/1
  MCU_IsMcuNOTActive_S/1 -> MCU_IsMcuNOTActivecv/1
  MCU_IsMcuNOTActive_L/1 -> MCU_IsMcuNOTActive_S/1
  MCU_IsMcuNOTActive_Convert/1 -> MCU_IsMcuNOTActive_L/1
  MCU_IsMcuNOTActive_Sub/1(Out1) -> MCU_IsMcuNOTActive_Convert/1
  Demux/5 -> MCU_IsFreeMode_Sub/1(In1), MCU_IsSpdMode_Sub/1(In1), MCU_IsBrakeMode_Sub/1(In1), MCU_IsMcuNOTActive_Sub/1(In1), MCU_IsTorqMode_Sub/1(In1), MCU_IsZeroLocMode_Sub/1(In1)
  MCU_IsMcuNOTActive_sat/1 -> MCU_IsMcuNOTActive_Out/1
  MCU_IsMcuNOTActive_Ad/1 -> MCU_IsMcuNOTActive_sat/1
  MCU_IsMcuNOTActive_O/1 -> MCU_IsMcuNOTActive_Ad/2
  MCU_IsMcuNOTActive_F/1 -> MCU_IsMcuNOTActive_Ad/1
  MCU_IsReadycv/1 -> MCU_IsReady_F/1
  MCU_IsReady_S/1 -> MCU_IsReadycv/1
  MCU_IsReady_L/1 -> MCU_IsReady_S/1
  MCU_IsReady_Convert/1 -> MCU_IsReady_L/1
  MCU_IsReady_Sub/1(Out1) -> MCU_IsReady_Convert/1
  MCU_IsReady_sat/1 -> MCU_IsReady_Out/1
  MCU_IsReady_Ad/1 -> MCU_IsReady_sat/1
  MCU_IsReady_O/1 -> MCU_IsReady_Ad/2
  MCU_IsReady_F/1 -> MCU_IsReady_Ad/1
  MCU_IsPreChgcv/1 -> MCU_IsPreChg_F/1
  MCU_IsPreChg_S/1 -> MCU_IsPreChgcv/1
  MCU_IsPreChg_L/1 -> MCU_IsPreChg_S/1
  MCU_IsPreChg_Convert/1 -> MCU_IsPreChg_L/1
  MCU_IsPreChg_Sub/1(Out1) -> MCU_IsPreChg_Convert/1
  MCU_IsPreChg_sat/1 -> MCU_IsPreChg_Out/1
  MCU_IsPreChg_Ad/1 -> MCU_IsPreChg_sat/1
  MCU_IsPreChg_O/1 -> MCU_IsPreChg_Ad/2
  MCU_IsPreChg_F/1 -> MCU_IsPreChg_Ad/1
  MCU_IsRevoloverErrorcv/1 -> MCU_IsRevoloverError_F/1
  MCU_IsRevoloverError_S/1 -> MCU_IsRevoloverErrorcv/1
  MCU_IsRevoloverError_L/1 -> MCU_IsRevoloverError_S/1
  MCU_IsRevoloverError_Convert/1 -> MCU_IsRevoloverError_L/1
  MCU_IsRevoloverError_Sub/1(Out1) -> MCU_IsRevoloverError_Convert/1
  MCU_IsRevoloverError_sat/1 -> MCU_IsRevoloverError_Out/1
  MCU_IsRevoloverError_Ad/1 -> MCU_IsRevoloverError_sat/1
  MCU_IsRevoloverError_O/1 -> MCU_IsRevoloverError_Ad/2
  MCU_IsRevoloverError_F/1 -> MCU_IsRevoloverError_Ad/1
  MCU_IsOverCurrcv/1 -> MCU_IsOverCurr_F/1
  MCU_IsOverCurr_S/1 -> MCU_IsOverCurrcv/1
  MCU_IsOverCurr_L/1 -> MCU_IsOverCurr_S/1
  MCU_IsOverCurr_Convert/1 -> MCU_IsOverCurr_L/1
  MCU_IsOverCurr_Sub/1(Out1) -> MCU_IsOverCurr_Convert/1
  MCU_IsOverCurr_sat/1 -> MCU_IsOverCurr_Out/1
  MCU_IsOverCurr_Ad/1 -> MCU_IsOverCurr_sat/1
  MCU_IsOverCurr_O/1 -> MCU_IsOverCurr_Ad/2
  MCU_IsOverCurr_F/1 -> MCU_IsOverCurr_Ad/1
  MCU_IsHvOvervoltagecv/1 -> MCU_IsHvOvervoltage_F/1
  MCU_IsHvOvervoltage_S/1 -> MCU_IsHvOvervoltagecv/1
  MCU_IsHvOvervoltage_L/1 -> MCU_IsHvOvervoltage_S/1
  MCU_IsHvOvervoltage_Convert/1 -> MCU_IsHvOvervoltage_L/1
  MCU_IsHvOvervoltage_Sub/1(Out1) -> MCU_IsHvOvervoltage_Convert/1
  MCU_IsHvOvervoltage_sat/1 -> MCU_IsHvOvervoltage_Out/1
  MCU_IsHvOvervoltage_Ad/1 -> MCU_IsHvOvervoltage_sat/1
  MCU_IsHvOvervoltage_O/1 -> MCU_IsHvOvervoltage_Ad/2
  MCU_IsHvOvervoltage_F/1 -> MCU_IsHvOvervoltage_Ad/1
  MCU_IsLvErrorcv/1 -> MCU_IsLvError_F/1
  MCU_IsLvError_S/1 -> MCU_IsLvErrorcv/1
  MCU_IsLvError_L/1 -> MCU_IsLvError_S/1
  MCU_IsLvError_Convert/1 -> MCU_IsLvError_L/1
  MCU_IsLvError_Sub/1(Out1) -> MCU_IsLvError_Convert/1
  MCU_IsLvError_sat/1 -> MCU_IsLvError_Out/1
  MCU_IsLvError_Ad/1 -> MCU_IsLvError_sat/1
  MCU_IsLvError_O/1 -> MCU_IsLvError_Ad/2
  MCU_IsLvError_F/1 -> MCU_IsLvError_Ad/1
  MCU_IsHvUndervoltagecv/1 -> MCU_IsHvUndervoltage_F/1
  MCU_IsHvUndervoltage_S/1 -> MCU_IsHvUndervoltagecv/1
  MCU_IsHvUndervoltage_L/1 -> MCU_IsHvUndervoltage_S/1
  MCU_IsHvUndervoltage_Convert/1 -> MCU_IsHvUndervoltage_L/1
  MCU_IsHvUndervoltage_Sub/1(Out1) -> MCU_IsHvUndervoltage_Convert/1
  MCU_IsHvUndervoltage_sat/1 -> MCU_IsHvUndervoltage_Out/1
  MCU_IsHvUndervoltage_Ad/1 -> MCU_IsHvUndervoltage_sat/1
  MCU_IsHvUndervoltage_O/1 -> MCU_IsHvUndervoltage_Ad/2
  MCU_IsHvUndervoltage_F/1 -> MCU_IsHvUndervoltage_Ad/1
  MCU_IsUnderPowerLimcv/1 -> MCU_IsUnderPowerLim_F/1
  MCU_IsUnderPowerLim_S/1 -> MCU_IsUnderPowerLimcv/1
  MCU_IsUnderPowerLim_L/1 -> MCU_IsUnderPowerLim_S/1
  MCU_IsUnderPowerLim_Convert/1 -> MCU_IsUnderPowerLim_L/1
  MCU_IsUnderPowerLim_Sub/1(Out1) -> MCU_IsUnderPowerLim_Convert/1
  Demux/6 -> MCU_IsHvUndervoltage_Sub/1(In1), MCU_IsUnderPowerLim_Sub/1(In1), MCU_IsLvError_Sub/1(In1), MCU_IsHvOvervoltage_Sub/1(In1), MCU_IsOverCurr_Sub/1(In1), MCU_IsRevoloverError_Sub/1(In1), MCU_IsPreChg_Sub/1(In1), MCU_IsReady_Sub/1(In1)
  MCU_IsUnderPowerLim_sat/1 -> MCU_IsUnderPowerLim_Out/1
  MCU_IsUnderPowerLim_Ad/1 -> MCU_IsUnderPowerLim_sat/1
  MCU_IsUnderPowerLim_O/1 -> MCU_IsUnderPowerLim_Ad/2
  MCU_IsUnderPowerLim_F/1 -> MCU_IsUnderPowerLim_Ad/1
  MCU_IsMcuOvertempcv/1 -> MCU_IsMcuOvertemp_F/1
  MCU_IsMcuOvertemp_S/1 -> MCU_IsMcuOvertempcv/1
  MCU_IsMcuOvertemp_L/1 -> MCU_IsMcuOvertemp_S/1
  MCU_IsMcuOvertemp_Convert/1 -> MCU_IsMcuOvertemp_L/1
  MCU_IsMcuOvertemp_Sub/1(Out1) -> MCU_IsMcuOvertemp_Convert/1
  MCU_IsMcuOvertemp_sat/1 -> MCU_IsMcuOvertemp_Out/1
  MCU_IsMcuOvertemp_Ad/1 -> MCU_IsMcuOvertemp_sat/1
  MCU_IsMcuOvertemp_O/1 -> MCU_IsMcuOvertemp_Ad/2
  MCU_IsMcuOvertemp_F/1 -> MCU_IsMcuOvertemp_Ad/1
  MCU_IsMotorOvertempcv/1 -> MCU_IsMotorOvertemp_F/1
  MCU_IsMotorOvertemp_S/1 -> MCU_IsMotorOvertempcv/1
  MCU_IsMotorOvertemp_L/1 -> MCU_IsMotorOvertemp_S/1
  MCU_IsMotorOvertemp_Convert/1 -> MCU_IsMotorOvertemp_L/1
  MCU_IsMotorOvertemp_Sub/1(Out1) -> MCU_IsMotorOvertemp_Convert/1
  MCU_IsMotorOvertemp_sat/1 -> MCU_IsMotorOvertemp_Out/1
  MCU_IsMotorOvertemp_Ad/1 -> MCU_IsMotorOvertemp_sat/1
  MCU_IsMotorOvertemp_O/1 -> MCU_IsMotorOvertemp_Ad/2
  MCU_IsMotorOvertemp_F/1 -> MCU_IsMotorOvertemp_Ad/1
  MCU_IsSelfcheckPasscv/1 -> MCU_IsSelfcheckPass_F/1
  MCU_IsSelfcheckPass_S/1 -> MCU_IsSelfcheckPasscv/1
  MCU_IsSelfcheckPass_L/1 -> MCU_IsSelfcheckPass_S/1
  MCU_IsSelfcheckPass_Convert/1 -> MCU_IsSelfcheckPass_L/1
  MCU_IsSelfcheckPass_Sub/1(Out1) -> MCU_IsSelfcheckPass_Convert/1
  Demux/7 -> MCU_IsMotorOvertemp_Sub/1(In1), MCU_IsSelfcheckPass_Sub/1(In1), MCU_IsMcuOvertemp_Sub/1(In1)
  MCU_IsSelfcheckPass_sat/1 -> MCU_IsSelfcheckPass_Out/1
  MCU_IsSelfcheckPass_Ad/1 -> MCU_IsSelfcheckPass_sat/1
  MCU_IsSelfcheckPass_O/1 -> MCU_IsSelfcheckPass_Ad/2
  MCU_IsSelfcheckPass_F/1 -> MCU_IsSelfcheckPass_Ad/1
  MCU_AlmLvcv/1 -> MCU_AlmLv_F/1
  MCU_AlmLv_S/1 -> MCU_AlmLvcv/1
  MCU_AlmLv_L/1 -> MCU_AlmLv_S/1
  MCU_AlmLv_Convert/1 -> MCU_AlmLv_L/1
  MCU_AlmLv_Sub/1(Out1) -> MCU_AlmLv_Convert/1
  Demux/8 -> MCU_AlmLv_Sub/1(In1)
  MCU_AlmLv_sat/1 -> MCU_AlmLv_Out/1
  MCU_AlmLv_Ad/1 -> MCU_AlmLv_sat/1
  MCU_AlmLv_O/1 -> MCU_AlmLv_Ad/2
  MCU_AlmLv_F/1 -> MCU_AlmLv_Ad/1

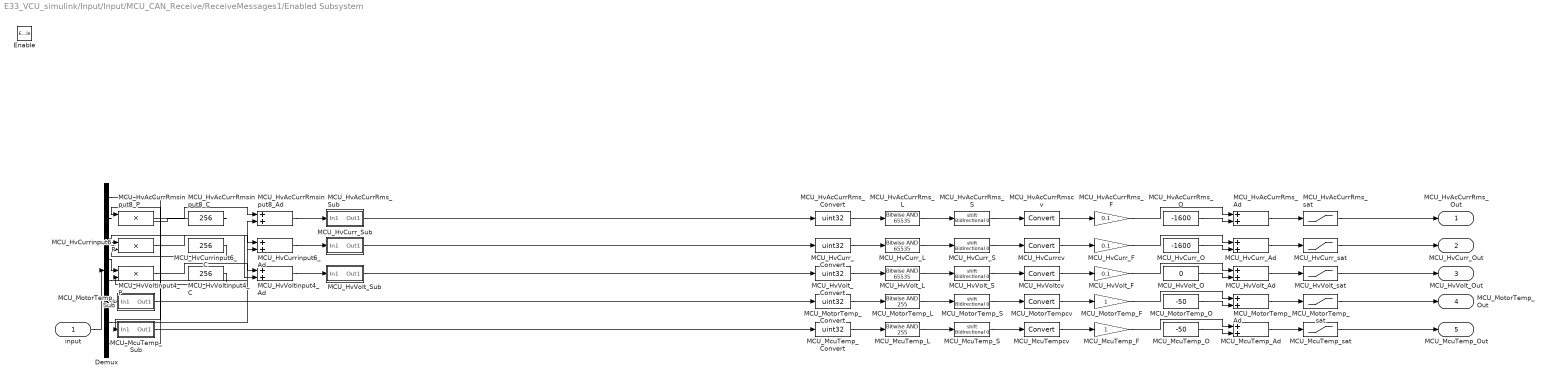
== system E33_VCU_simulink/Input/Input/MCU_CAN_Receive/ReceiveMessages1/Enabled Subsystem ==
  input : Inport
  Enable : EnablePort
  Demux : Demux  Outputs=8
  MCU_HvAcCurrRms_Ad : Sum
  MCU_HvAcCurrRms_Convert : DataTypeConversion  OutDataTypeStr=uint32
  MCU_HvAcCurrRms_F : Gain  Gain=0.1
  MCU_HvAcCurrRms_L : simulink/Logic and Bit Operations/Bitwise Operator  logicop=AND  UseBitMask=on  BitMask=65535  BitMaskRealWorld=Stored Integer
  MCU_HvAcCurrRms_O : Constant  Value=-1600  OutDataTypeStr=single
  MCU_HvAcCurrRms_S : ArithShift
  MCU_HvAcCurrRms_Sub : Subsystem
  MCU_HvAcCurrRms_sat : Saturate  UpperLimit=1600  LowerLimit=-1600
  MCU_HvAcCurrRmscv : DataTypeConversion
  MCU_HvAcCurrRmsinput8_Ad : Sum
  MCU_HvAcCurrRmsinput8_C : Constant  Value=256
  MCU_HvAcCurrRmsinput8_P : Product
  MCU_HvCurr_Ad : Sum
  MCU_HvCurr_Convert : DataTypeConversion  OutDataTypeStr=uint32
  MCU_HvCurr_F : Gain  Gain=0.1
  MCU_HvCurr_L : simulink/Logic and Bit Operations/Bitwise Operator  logicop=AND  UseBitMask=on  BitMask=65535  BitMaskRealWorld=Stored Integer
  MCU_HvCurr_O : Constant  Value=-1600  OutDataTypeStr=single
  MCU_HvCurr_S : ArithShift
  MCU_HvCurr_Sub : Subsystem
  MCU_HvCurr_sat : Saturate  UpperLimit=1600  LowerLimit=-1600
  MCU_HvCurrcv : DataTypeConversion
  MCU_HvCurrinput6_Ad : Sum
  MCU_HvCurrinput6_C : Constant  Value=256
  MCU_HvCurrinput6_P : Product
  MCU_HvVolt_Ad : Sum
  MCU_HvVolt_Convert : DataTypeConversion  OutDataTypeStr=uint32
  MCU_HvVolt_F : Gain  Gain=0.1
  MCU_HvVolt_L : simulink/Logic and Bit Operations/Bitwise Operator  logicop=AND  UseBitMask=on  BitMask=65535  BitMaskRealWorld=Stored Integer
  MCU_HvVolt_O : Constant  Value=0  OutDataTypeStr=single
  MCU_HvVolt_S : ArithShift
  MCU_HvVolt_Sub : Subsystem
  MCU_HvVolt_sat : Saturate  UpperLimit=1000  LowerLimit=0
  MCU_HvVoltcv : DataTypeConversion
  MCU_HvVoltinput4_Ad : Sum
  MCU_HvVoltinput4_C : Constant  Value=256
  MCU_HvVoltinput4_P : Product
  MCU_McuTemp_Ad : Sum
  MCU_McuTemp_Convert : DataTypeConversion  OutDataTypeStr=uint32
  MCU_McuTemp_F : Gain
  MCU_McuTemp_L : simulink/Logic and Bit Operations/Bitwise Operator  logicop=AND  UseBitMask=on  BitMask=255  BitMaskRealWorld=Stored Integer
  MCU_McuTemp_O : Constant  Value=-50  OutDataTypeStr=single
  MCU_McuTemp_S : ArithShift
  MCU_McuTemp_Sub : Subsystem
  MCU_McuTemp_sat : Saturate  UpperLimit=205  LowerLimit=-50
  MCU_McuTempcv : DataTypeConversion
  MCU_MotorTemp_Ad : Sum
  MCU_MotorTemp_Convert : DataTypeConversion  OutDataTypeStr=uint32
  MCU_MotorTemp_F : Gain
  MCU_MotorTemp_L : simulink/Logic and Bit Operations/Bitwise Operator  logicop=AND  UseBitMask=on  BitMask=255  BitMaskRealWorld=Stored Integer
  MCU_MotorTemp_O : Constant  Value=-50  OutDataTypeStr=single
  MCU_MotorTemp_S : ArithShift
  MCU_MotorTemp_Sub : Subsystem
  MCU_MotorTemp_sat : Saturate  UpperLimit=205  LowerLimit=-50
  MCU_MotorTempcv : DataTypeConversion
  MCU_HvAcCurrRms_Out : Outport
  MCU_HvCurr_Out : Outport  Port=2
  MCU_HvVolt_Out : Outport  Port=3
  MCU_MotorTemp_Out : Outport  Port=4
  MCU_McuTemp_Out : Outport  Port=5
  wires:
  MCU_HvAcCurrRms_F/1 -> MCU_HvAcCurrRms_Ad/1
  MCU_HvAcCurrRms_O/1 -> MCU_HvAcCurrRms_Ad/2
  MCU_HvAcCurrRms_Ad/1 -> MCU_HvAcCurrRms_sat/1
  MCU_HvAcCurrRms_sat/1 -> MCU_HvAcCurrRms_Out/1
  Demux/8 -> MCU_HvAcCurrRmsinput8_P/1
  MCU_HvAcCurrRmsinput8_C/1 -> MCU_HvAcCurrRmsinput8_P/2
  MCU_HvAcCurrRmsinput8_P/1 -> MCU_HvAcCurrRmsinput8_Ad/1
  Demux/7 -> MCU_HvAcCurrRmsinput8_Ad/2
  MCU_HvAcCurrRmsinput8_Ad/1 -> MCU_HvAcCurrRms_Sub/1(In1)
  MCU_HvAcCurrRms_Sub/1(Out1) -> MCU_HvAcCurrRms_Convert/1
  MCU_HvAcCurrRms_Convert/1 -> MCU_HvAcCurrRms_L/1
  MCU_HvAcCurrRms_L/1 -> MCU_HvAcCurrRms_S/1
  MCU_HvAcCurrRms_S/1 -> MCU_HvAcCurrRmscv/1
  MCU_HvAcCurrRmscv/1 -> MCU_HvAcCurrRms_F/1
  MCU_HvCurr_F/1 -> MCU_HvCurr_Ad/1
  MCU_HvCurr_O/1 -> MCU_HvCurr_Ad/2
  MCU_HvCurr_Ad/1 -> MCU_HvCurr_sat/1
  MCU_HvCurr_sat/1 -> MCU_HvCurr_Out/1
  Demux/6 -> MCU_HvCurrinput6_P/1
  MCU_HvCurrinput6_C/1 -> MCU_HvCurrinput6_P/2
  MCU_HvCurrinput6_P/1 -> MCU_HvCurrinput6_Ad/1
  Demux/5 -> MCU_HvCurrinput6_Ad/2
  MCU_HvCurrinput6_Ad/1 -> MCU_HvCurr_Sub/1(In1)
  MCU_HvCurr_Sub/1(Out1) -> MCU_HvCurr_Convert/1
  MCU_HvCurr_Convert/1 -> MCU_HvCurr_L/1
  MCU_HvCurr_L/1 -> MCU_HvCurr_S/1
  MCU_HvCurr_S/1 -> MCU_HvCurrcv/1
  MCU_HvCurrcv/1 -> MCU_HvCurr_F/1
  MCU_HvVolt_F/1 -> MCU_HvVolt_Ad/1
  MCU_HvVolt_O/1 -> MCU_HvVolt_Ad/2
  MCU_HvVolt_Ad/1 -> MCU_HvVolt_sat/1
  MCU_HvVolt_sat/1 -> MCU_HvVolt_Out/1
  Demux/4 -> MCU_HvVoltinput4_P/1
  MCU_HvVoltinput4_C/1 -> MCU_HvVoltinput4_P/2
  MCU_HvVoltinput4_P/1 -> MCU_HvVoltinput4_Ad/1
  Demux/3 -> MCU_HvVoltinput4_Ad/2
  MCU_HvVoltinput4_Ad/1 -> MCU_HvVolt_Sub/1(In1)
  MCU_HvVolt_Sub/1(Out1) -> MCU_HvVolt_Convert/1
  MCU_HvVolt_Convert/1 -> MCU_HvVolt_L/1
  MCU_HvVolt_L/1 -> MCU_HvVolt_S/1
  MCU_HvVolt_S/1 -> MCU_HvVoltcv/1
  MCU_HvVoltcv/1 -> MCU_HvVolt_F/1
  MCU_MotorTemp_F/1 -> MCU_MotorTemp_Ad/1
  MCU_MotorTemp_O/1 -> MCU_MotorTemp_Ad/2
  MCU_MotorTemp_Ad/1 -> MCU_MotorTemp_sat/1
  MCU_MotorTemp_sat/1 -> MCU_MotorTemp_Out/1
  Demux/2 -> MCU_MotorTemp_Sub/1(In1)
  MCU_MotorTemp_Sub/1(Out1) -> MCU_MotorTemp_Convert/1
  MCU_MotorTemp_Convert/1 -> MCU_MotorTemp_L/1
  MCU_MotorTemp_L/1 -> MCU_MotorTemp_S/1
  MCU_MotorTemp_S/1 -> MCU_MotorTempcv/1
  MCU_MotorTempcv/1 -> MCU_MotorTemp_F/1
  MCU_McuTemp_F/1 -> MCU_McuTemp_Ad/1
  MCU_McuTemp_O/1 -> MCU_McuTemp_Ad/2
  MCU_McuTemp_Ad/1 -> MCU_McuTemp_sat/1
  MCU_McuTemp_sat/1 -> MCU_McuTemp_Out/1
  Demux/1 -> MCU_McuTemp_Sub/1(In1)
  MCU_McuTemp_Sub/1(Out1) -> MCU_McuTemp_Convert/1
  MCU_McuTemp_Convert/1 -> MCU_McuTemp_L/1
  MCU_McuTemp_L/1 -> MCU_McuTemp_S/1
  MCU_McuTemp_S/1 -> MCU_McuTempcv/1
  MCU_McuTempcv/1 -> MCU_McuTemp_F/1
  input/1 -> Demux/1

== system E33_VCU_simulink/Input/Input/Sensor/For Each Subsystem/Filter5 ==
  In : Inport
  Add : Sum  Inputs=-+-
  Constant : Constant  Value=4  OutDataTypeStr=uint8  SampleTime=-1
  Divide : Product  Inputs=*/
  MinMax : MinMax
  MinMax1 : MinMax  Function=max
  Sum of Elements : Sum  Inputs=+
  Tapped Delay : simulink/Discrete/Tapped Delay  vinit=0  samptime=-1  NumDelays=6  DelayOrder=Oldest  includeCurrent=off
  Out : Outport
  wires:
  Constant/1 -> Divide/2
  Sum of Elements/1 -> Add/2
  MinMax1/1 -> Add/1
  MinMax/1 -> Add/3
  Add/1 -> Divide/1
  In/1 -> Tapped Delay/1
  Divide/1 -> Out/1
  Tapped Delay/1 -> Sum of Elements/1, MinMax1/1, MinMax/1

== system E33_VCU_simulink/Input/Input/BMS_CAN_Receive/BMS_ALM_Analyze/Enabled Subsystem/BMS_ALM_AUX_FAIL_Sub ==
  In1 : Inport
  Out1 : Outport
  wires:
  In1/1 -> Out1/1

== system E33_VCU_simulink/Input/Input/BMS_CAN_Receive/BMS_ALM_Analyze/Enabled Subsystem/BMS_ALM_BATT_OC_Sub ==
  In1 : Inport
  Out1 : Outport
  wires:
  In1/1 -> Out1/1

== system E33_VCU_simulink/Input/Input/BMS_CAN_Receive/BMS_ALM_Analyze/Enabled Subsystem/BMS_ALM_BATT_OV_Sub ==
  In1 : Inport
  Out1 : Outport
  wires:
  In1/1 -> Out1/1

== system E33_VCU_simulink/Input/Input/BMS_CAN_Receive/BMS_ALM_Analyze/Enabled Subsystem/BMS_ALM_BATT_UC_Sub ==
  In1 : Inport
  Out1 : Outport
  wires:
  In1/1 -> Out1/1

== system E33_VCU_simulink/Input/Input/BMS_CAN_Receive/BMS_ALM_Analyze/Enabled Subsystem/BMS_ALM_BATT_UV_Sub ==
  In1 : Inport
  Out1 : Outport
  wires:
  In1/1 -> Out1/1

== system E33_VCU_simulink/Input/Input/BMS_CAN_Receive/BMS_ALM_Analyze/Enabled Subsystem/BMS_ALM_BMU_FAIL_Sub ==
  In1 : Inport
  Out1 : Outport
  wires:
  In1/1 -> Out1/1

== system E33_VCU_simulink/Input/Input/BMS_CAN_Receive/BMS_ALM_Analyze/Enabled Subsystem/BMS_ALM_BSU_FAULT_Sub ==
  In1 : Inport
  Out1 : Outport
  wires:
  In1/1 -> Out1/1

== system E33_VCU_simulink/Input/Input/BMS_CAN_Receive/BMS_ALM_Analyze/Enabled Subsystem/BMS_ALM_BSU_OFFLINE_Sub ==
  In1 : Inport
  Out1 : Outport
  wires:
  In1/1 -> Out1/1

== system E33_VCU_simulink/Input/Input/BMS_CAN_Receive/BMS_ALM_Analyze/Enabled Subsystem/BMS_ALM_CELL_DT_Sub ==
  In1 : Inport
  Out1 : Outport
  wires:
  In1/1 -> Out1/1

== system E33_VCU_simulink/Input/Input/BMS_CAN_Receive/BMS_ALM_Analyze/Enabled Subsystem/BMS_ALM_CELL_DV_Sub ==
  In1 : Inport
  Out1 : Outport
  wires:
  In1/1 -> Out1/1

== system E33_VCU_simulink/Input/Input/BMS_CAN_Receive/BMS_ALM_Analyze/Enabled Subsystem/BMS_ALM_CELL_LBK_Sub ==
  In1 : Inport
  Out1 : Outport
  wires:
  In1/1 -> Out1/1

== system E33_VCU_simulink/Input/Input/BMS_CAN_Receive/BMS_ALM_Analyze/Enabled Subsystem/BMS_ALM_CELL_OT_Sub ==
  In1 : Inport
  Out1 : Outport
  wires:
  In1/1 -> Out1/1

== system E33_VCU_simulink/Input/Input/BMS_CAN_Receive/BMS_ALM_Analyze/Enabled Subsystem/BMS_ALM_CELL_OV_Sub ==
  In1 : Inport
  Out1 : Outport
  wires:
  In1/1 -> Out1/1

== system E33_VCU_simulink/Input/Input/BMS_CAN_Receive/BMS_ALM_Analyze/Enabled Subsystem/BMS_ALM_CELL_TBK_Sub ==
  In1 : Inport
  Out1 : Outport
  wires:
  In1/1 -> Out1/1

== system E33_VCU_simulink/Input/Input/BMS_CAN_Receive/BMS_ALM_Analyze/Enabled Subsystem/BMS_ALM_CELL_UT_Sub ==
  In1 : Inport
  Out1 : Outport
  wires:
  In1/1 -> Out1/1

== system E33_VCU_simulink/Input/Input/BMS_CAN_Receive/BMS_ALM_Analyze/Enabled Subsystem/BMS_ALM_CELL_UV_Sub ==
  In1 : Inport
  Out1 : Outport
  wires:
  In1/1 -> Out1/1

== system E33_VCU_simulink/Input/Input/BMS_CAN_Receive/BMS_ALM_Analyze/Enabled Subsystem/BMS_ALM_CHRG_OCS_Sub ==
  In1 : Inport
  Out1 : Outport
  wires:
  In1/1 -> Out1/1

== system E33_VCU_simulink/Input/Input/BMS_CAN_Receive/BMS_ALM_Analyze/Enabled Subsystem/BMS_ALM_CHRG_OCT_Sub ==
  In1 : Inport
  Out1 : Outport
  wires:
  In1/1 -> Out1/1

== system E33_VCU_simulink/Input/Input/BMS_CAN_Receive/BMS_ALM_Analyze/Enabled Subsystem/BMS_ALM_DSCH_OCS_Sub ==
  In1 : Inport
  Out1 : Outport
  wires:
  In1/1 -> Out1/1

== system E33_VCU_simulink/Input/Input/BMS_CAN_Receive/BMS_ALM_Analyze/Enabled Subsystem/BMS_ALM_DSCH_OCT_Sub ==
  In1 : Inport
  Out1 : Outport
  wires:
  In1/1 -> Out1/1

== system E33_VCU_simulink/Input/Input/BMS_CAN_Receive/BMS_ALM_Analyze/Enabled Subsystem/BMS_ALM_HALL_BREAK_Sub ==
  In1 : Inport
  Out1 : Outport
  wires:
  In1/1 -> Out1/1

== system E33_VCU_simulink/Input/Input/BMS_CAN_Receive/BMS_ALM_Analyze/Enabled Subsystem/BMS_ALM_HVREL_FAIL_Sub ==
  In1 : Inport
  Out1 : Outport
  wires:
  In1/1 -> Out1/1

== system E33_VCU_simulink/Input/Input/BMS_CAN_Receive/BMS_ALM_Analyze/Enabled Subsystem/BMS_ALM_LEAK_OC_Sub ==
  In1 : Inport
  Out1 : Outport
  wires:
  In1/1 -> Out1/1

== system E33_VCU_simulink/Input/Input/BMS_CAN_Receive/BMS_ALM_Analyze/Enabled Subsystem/BMS_ALM_PRECHG_FAIL_Sub ==
  In1 : Inport
  Out1 : Outport
  wires:
  In1/1 -> Out1/1

== system E33_VCU_simulink/Input/Input/BMS_CAN_Receive/BMS_ALM_Analyze/Enabled Subsystem/BMS_ALM_VCU_OFFLINE_Sub ==
  In1 : Inport
  Out1 : Outport
  wires:
  In1/1 -> Out1/1

== system E33_VCU_simulink/Input/Input/BMS_CAN_Receive/BMS_ALM_Analyze1/BMS_HCU_MAXV/MaxCellVoltNo_Sub ==
  In1 : Inport
  Out1 : Outport
  wires:
  In1/1 -> Out1/1

== system E33_VCU_simulink/Input/Input/BMS_CAN_Receive/BMS_ALM_Analyze1/BMS_HCU_MAXV/MaxCellVolt_Sub ==
  In1 : Inport
  Out1 : Outport
  wires:
  In1/1 -> Out1/1

== system E33_VCU_simulink/Input/Input/BMS_CAN_Receive/BMS_ALM_Analyze1/BMS_HCU_MAXV/MinCellVoltNo_Sub ==
  In1 : Inport
  Out1 : Outport
  wires:
  In1/1 -> Out1/1

== system E33_VCU_simulink/Input/Input/BMS_CAN_Receive/BMS_ALM_Analyze1/BMS_HCU_MAXV/MinCellVolt_Sub ==
  In1 : Inport
  Out1 : Outport
  wires:
  In1/1 -> Out1/1

== system E33_VCU_simulink/Input/Input/BMS_CAN_Receive/BMS_INFO_Analyze/Enabled Subsystem/BatAlmLv_Sub ==
  In1 : Inport
  Out1 : Outport
  wires:
  In1/1 -> Out1/1

== system E33_VCU_simulink/Input/Input/BMS_CAN_Receive/BMS_INFO_Analyze/Enabled Subsystem/BatCurrent_Sub ==
  In1 : Inport
  Out1 : Outport
  wires:
  In1/1 -> Out1/1

== system E33_VCU_simulink/Input/Input/BMS_CAN_Receive/BMS_INFO_Analyze/Enabled Subsystem/BatLife_Sub ==
  In1 : Inport
  Out1 : Outport
  wires:
  In1/1 -> Out1/1

== system E33_VCU_simulink/Input/Input/BMS_CAN_Receive/BMS_INFO_Analyze/Enabled Subsystem/BatSoc_Sub ==
  In1 : Inport
  Out1 : Outport
  wires:
  In1/1 -> Out1/1

== system E33_VCU_simulink/Input/Input/BMS_CAN_Receive/BMS_INFO_Analyze/Enabled Subsystem/BatSoh_Sub ==
  In1 : Inport
  Out1 : Outport
  wires:
  In1/1 -> Out1/1

== system E33_VCU_simulink/Input/Input/BMS_CAN_Receive/BMS_INFO_Analyze/Enabled Subsystem/BatState_Sub ==
  In1 : Inport
  Out1 : Outport
  wires:
  In1/1 -> Out1/1

== system E33_VCU_simulink/Input/Input/BMS_CAN_Receive/BMS_INFO_Analyze/Enabled Subsystem/BatVoltage_Sub ==
  In1 : Inport
  Out1 : Outport
  wires:
  In1/1 -> Out1/1

== system E33_VCU_simulink/Input/Input/BMS_CAN_Receive/BMS_MAXT_Analyze/Enabled Subsystem/CoolingCtl_Sub ==
  In1 : Inport
  Out1 : Outport
  wires:
  In1/1 -> Out1/1

== system E33_VCU_simulink/Input/Input/BMS_CAN_Receive/BMS_MAXT_Analyze/Enabled Subsystem/HeatingCtl_Sub ==
  In1 : Inport
  Out1 : Outport
  wires:
  In1/1 -> Out1/1

== system E33_VCU_simulink/Input/Input/BMS_CAN_Receive/BMS_MAXT_Analyze/Enabled Subsystem/MaxTempNo_Sub ==
  In1 : Inport
  Out1 : Outport
  wires:
  In1/1 -> Out1/1

== system E33_VCU_simulink/Input/Input/BMS_CAN_Receive/BMS_MAXT_Analyze/Enabled Subsystem/MaxTemp_Sub ==
  In1 : Inport
  Out1 : Outport
  wires:
  In1/1 -> Out1/1

== system E33_VCU_simulink/Input/Input/BMS_CAN_Receive/BMS_MAXT_Analyze/Enabled Subsystem/MinTempNo_Sub ==
  In1 : Inport
  Out1 : Outport
  wires:
  In1/1 -> Out1/1

== system E33_VCU_simulink/Input/Input/BMS_CAN_Receive/BMS_MAXT_Analyze/Enabled Subsystem/MinTemp_Sub ==
  In1 : Inport
  Out1 : Outport
  wires:
  In1/1 -> Out1/1

== system E33_VCU_simulink/Input/Input/MCU_CAN_Receive/ReceiveMessages/MCU_Stat/MCU_AlmLv_Sub ==
  In1 : Inport
  Out1 : Outport
  wires:
  In1/1 -> Out1/1

== system E33_VCU_simulink/Input/Input/MCU_CAN_Receive/ReceiveMessages/MCU_Stat/MCU_IsBrakeMode_Sub ==
  In1 : Inport
  Out1 : Outport
  wires:
  In1/1 -> Out1/1
